simulink model "tests_control_franka"  (R2020b)
settings: Solver=ode1  StartTime=0.0  StopTime=5  FixedStep=0.001  RelTol=1e-4
values from neighbouring files (symbols this model uses):
  a0 = 0.99    [init.m]
  berta = 0.98    [init.m]
  csi = 1    [init.m]
  e_max = 0.01    [init.m]
  F_int_max = 5    [init.m]
  F_max = 2    [init.m]
  M = 1    [init.m]
  mass = 1    [init.m]
  q_max = q_max - deg2rad([0 0 0 10 0 5 0])    [init.m]
  q_min = q_min + deg2rad([0 0 0 10 0 5 0])    [init.m]
libraries: simulink x4
(part 1 of 2)
settings Model: Creator=Rachele  LastModifiedBy=giorg

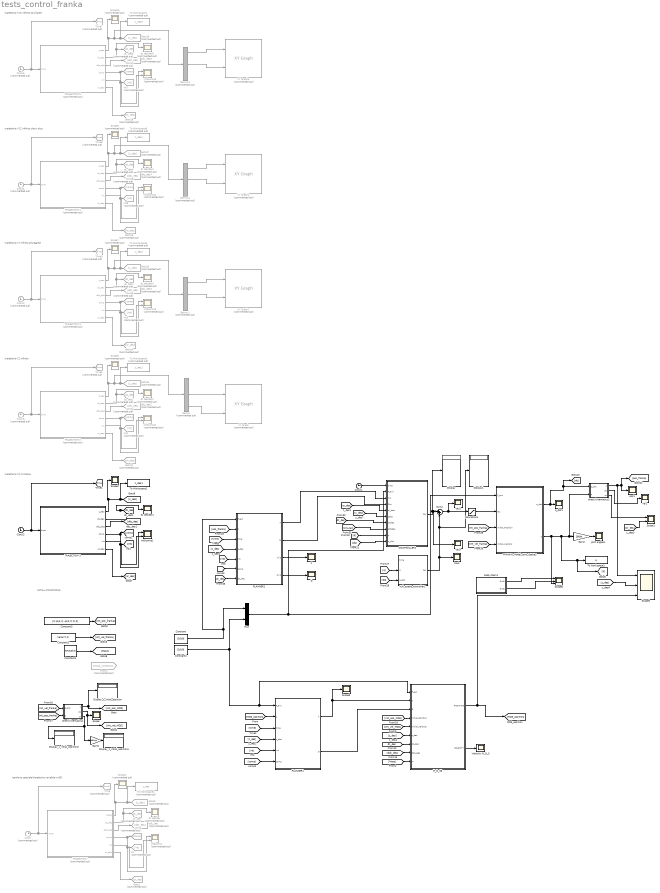
== system tests_control_franka ==
  note: bambino speciale(traiettoria variabile in 6D)
  note: INITIAL CONDITIONS
  note: traiettoria YZ circolare
  note: traiettoria YZ infinito
  note: traiettoria XY infinito allungante
  note: traiettoria XYZ infinito che si alza
  note: traiettoria XYZ infinito oscillante
  CONTROLLER1 : MATLAB Function  TreatAsAtomicUnit=on
  Clock{,3..6} (5 alike) : Clock  Commented=on
  Clock1 : Clock
  Clock2 : Clock
  Constant : Constant  Value=[0;0;0]
  Constant1 : Constant  Value=[0;0;0]
  Constant2 : Constant  Value=zeros(7,1)
  Constant3 : Constant  Value=[0; pi/4; 0; -pi/2; 0; 0; 0]  VectorParams1D=off
  Constant4 : Constant  Value=M*eye(3)
  D : Scope
  Demux{,1..3} (4 alike) : Demux  Commented=on  Outputs=3
  Display : Display
  Display1 : Display
  Display_z_intial_position : Display
  Display_z_intial_position1 : Display
  Display_z_intial_position2 : Display
  FRANKA_Model_Joint_Space2 : Subsystem
  From4 : From  Commented=on  GotoTag=initial_condition
  Gain2 : Gain  Gain=180/pi
  Gain3 : Gain  Gain=180/pi
  Goto{1,12,14,16,18} (5 alike) : Goto  Commented=on  GotoTag=or_des
  Goto{6,13,15,17,19} (5 alike) : Goto  Commented=on  GotoTag=z_des
  Joint angles1 : Scope
  K : Scope
  M_D_S5 : Subsystem
  Mux : Mux  Inputs=2
  PLANNER1 : Subsystem
  PLANNER2 : Subsystem
  Saturation1 : Saturate  UpperLimit=100  LowerLimit=-100
  Scope : Scope
  Scope1 : Scope  NumInputPorts=2
  Scope{4..5,7,9..10} (5 alike) : Scope  Commented=on
  Scope2 : Scope
  Scope3 : Scope
  Scope6 : Scope  NumInputPorts=3
  Scope8 : Scope  NumInputPorts=3
  Subsystem1 : Subsystem
  Sum2 : Sum  Inputs=|++
  TRAJECTORY : Subsystem  Commented=on
  TRAJECTORY1 : Subsystem
  TRAJECTORY2 : Subsystem  Commented=on
  TRAJECTORY3 : Subsystem  Commented=on
  TRAJECTORY4 : Subsystem  Commented=on
  TRAJECTORY5 : Subsystem  Commented=on
  Time{,4..7} (5 alike) : Goto  Commented=on  GotoTag=time
  To Workspace1 : ToWorkspace  VariableName=q  SaveFormat=Timeseries  SampleTime=-1
  To Workspace2 : ToWorkspace  VariableName=z_des1  SaveFormat=Timeseries  SampleTime=-1
      settings: Save2DSignal=2-D array (concatenate along first dimension)
  To Workspace3 : ToWorkspace  Commented=on  VariableName=z_des2  SaveFormat=Timeseries  SampleTime=-1
      settings: Save2DSignal=2-D array (concatenate along first dimension)
  To Workspace4 : ToWorkspace  Commented=on  VariableName=z_des  SaveFormat=Timeseries  SampleTime=-1
      settings: Save2DSignal=2-D array (concatenate along first dimension)
  To Workspace5 : ToWorkspace  Commented=on  VariableName=z_des3  SaveFormat=Timeseries  SampleTime=-1
      settings: Save2DSignal=2-D array (concatenate along first dimension)
  To Workspace6 : ToWorkspace  Commented=on  VariableName=z_des4  SaveFormat=Timeseries  SampleTime=-1
      settings: Save2DSignal=2-D array (concatenate along first dimension)
  To Workspace7 : ToWorkspace  Commented=on  VariableName=z_des5  SaveFormat=Timeseries  SampleTime=-1
      settings: Save2DSignal=2-D array (concatenate along first dimension)
  Velocity M_D_S : Scope
  XY Graph{,1..3} (4 alike) : simulink/Sinks/XY Graph  Commented=on  xmin=-1/2  xmax=1/2  ymin=-1/2  ymax=1/2  st=-1
  comp{,4..7} (5 alike) : Goto  Commented=on  GotoTag=comp
  ddz_des{,2..5} (5 alike) : Goto  Commented=on  GotoTag=ddz_des
  direct kinematics1 : MATLAB Function  TreatAsAtomicUnit=on
  direct kinematics2 : MATLAB Function  TreatAsAtomicUnit=on
  dz desider{,2..5} (5 alike) : Scope  Commented=on
  dz desider1 : Scope
  dz_des{,2..5} (5 alike) : Goto  Commented=on  GotoTag=dz_des  TagVisibility=global
  int{,4..7} (5 alike) : Goto  Commented=on  GotoTag=int
  int&comp{,2..5} (5 alike) : Scope  Commented=on  NumInputPorts=2
  int&comp1 : Scope  NumInputPorts=2
  null_space_controller1 : MATLAB Function  TreatAsAtomicUnit=on
  pos1 : Scope
  q_dot1 : Scope
  tau1 : Scope
  tau2 : Scope
  tau3 : Scope
  vel1 : Scope
  tag scope: dz_des=global
  wires:
  TRAJECTORY/1(z_des) -> Goto6/1, To Workspace4/1, Scope4/1
  [int] -> PLANNER1/5(int)
  PLANNER1/1(K) -> M_D_S5/2(K), Scope3/1
  [init_vel_franka] -> direct kinematics1/1(q_dot)
  Constant3/1 -> [init_pos_franka]
  [MDS_position] -> PLANNER1/2(z)
  Clock/1 -> TRAJECTORY/1(time), Time/1
  [init_vel_MDS] -> M_D_S5/5(Initial_Velocity)
  direct kinematics1/1(z) -> [init_pos_MDS], Display_z_intial_position/1
  Constant4/1 -> [Mass]
  TRAJECTORY/5(int) -> int&comp/2, int/1
  [init_pos_franka] -> direct kinematics1/2(q)
  [dz_des] -> M_D_S5/7(dz_des)
  [z_des] -> PLANNER1/4(z_des)
  [comp] -> PLANNER1/6(comp)
  [ddz_des] -> M_D_S5/8(ddz_des)
  M_D_S5/2(VELOCITY) -> Velocity M_D_S/1
  TRAJECTORY/4(comp) -> int&comp/1, comp/1
  [time] -> PLANNER1/3(time)
  TRAJECTORY/3(ddz_des) -> ddz_des/1
  [Mass] -> M_D_S5/9(M)
  [init_pos_MDS] -> M_D_S5/4(Initial_Position)
  TRAJECTORY/2(dz_des) -> dz desider/1, dz_des/1
  Constant2/1 -> [init_vel_franka]
  [z_des] -> M_D_S5/6(z_des)
  M_D_S5/1(POSITION) -> Scope8/3, [MDS_position]
  [comp] -> PLANNER2/6(comp)
  Subsystem1/1(Out1) -> Scope6/1
  direct kinematics2/3(or) -> Scope1/1
  [or_des] -> CONTROLLER1/5(or_des)
  [dq] -> CONTROLLER1/10(q_dot)
  direct kinematics2/2(dz) -> vel1/1
  [ddz_des] -> CONTROLLER1/8(ddzdes)
  [z_des] -> PLANNER2/4(z_des)
  Gain2/1 -> Joint angles1/1
  [dq] -> null_space_controller1/3(q_dot)
  [time] -> PLANNER2/3(time)
  [pos_franka] -> PLANNER2/2(z)
  [init_pos_franka] -> FRANKA_Model_Joint_Space2/3(Initial_Position)
  FRANKA_Model_Joint_Space2/1(q_dot) -> [dq], direct kinematics2/1(q_dot), q_dot1/1
  direct kinematics2/1(z) -> Scope8/1, pos1/1, [pos_franka]
  [int] -> PLANNER2/5(int)
  [z_des] -> Scope8/2
  [z_des] -> CONTROLLER1/6(zdes)
  null_space_controller1/1(tau) -> tau2/1, Display1/1, Sum2/2
  Sum2/1 -> Saturation1/1, tau1/1
  PLANNER2/1(K) -> CONTROLLER1/3(Km)
  FRANKA_Model_Joint_Space2/2(q) -> Scope6/3, [q], To Workspace1/1, direct kinematics2/2(q), Gain2/1
  [dz_des] -> CONTROLLER1/7(dzdes)
  [q] -> null_space_controller1/2(q)
  PLANNER2/2(D) -> CONTROLLER1/4(Dm)
  [init_vel_franka] -> FRANKA_Model_Joint_Space2/4(Initial_Velocity)
  CONTROLLER1/1(tau) -> Display/1, tau3/1, Sum2/1
  Saturation1/1 -> FRANKA_Model_Joint_Space2/2(tau)
  Subsystem1/2(Out2) -> Scope6/2
  [q] -> CONTROLLER1/9(q)
  PLANNER1/2(D) -> M_D_S5/3(D)
  direct kinematics1/2(dz) -> Scope/1, [init_vel_MDS]
  Gain3/1 -> Display_z_intial_position1/1
  direct kinematics1/3(or) -> Gain3/1, Display_z_intial_position2/1
  PLANNER2/3(kvis) -> K/1
  PLANNER2/4(dvis) -> D/1
  [dz_des] -> PLANNER2/7(dz_des)
  Constant/1 -> Mux/1, PLANNER2/1(F_ext)
  Constant1/1 -> M_D_S5/1(F_ext), PLANNER1/1(F_ext), Mux/2
  Mux/1 -> CONTROLLER1/2(F_ext), FRANKA_Model_Joint_Space2/1(F_ext)
  TRAJECTORY/6(or_des) -> Goto1/1
  Clock1/1 -> CONTROLLER1/1(time)
  [or_des] -> Scope1/2
  TRAJECTORY1/6(or_des) -> [or_des]
  TRAJECTORY1/2(dz_des) -> dz desider1/1, [dz_des]
  TRAJECTORY1/3(ddz_des) -> [ddz_des]
  TRAJECTORY1/4(comp) -> [comp], int&comp1/1
  TRAJECTORY1/5(int) -> [int], int&comp1/2
  Clock2/1 -> [time], TRAJECTORY1/1(time)
  TRAJECTORY1/1(z_des) -> Scope2/1, To Workspace2/1, [z_des]
  Clock3/1 -> Time4/1, TRAJECTORY2/1(time)
  TRAJECTORY2/1(z_des) -> Scope5/1, Demux/1, To Workspace3/1, Goto13/1
  TRAJECTORY2/5(int) -> int4/1, int&comp2/2
  TRAJECTORY2/4(comp) -> comp4/1, int&comp2/1
  TRAJECTORY2/6(or_des) -> Goto12/1
  TRAJECTORY2/2(dz_des) -> dz_des2/1, dz desider2/1
  TRAJECTORY2/3(ddz_des) -> ddz_des2/1
  Demux/2 -> XY Graph/1
  Demux/3 -> XY Graph/2
  TRAJECTORY3/3(ddz_des) -> ddz_des3/1
  TRAJECTORY3/2(dz_des) -> dz_des3/1, dz desider3/1
  TRAJECTORY3/6(or_des) -> Goto14/1
  TRAJECTORY3/4(comp) -> comp5/1, int&comp3/1
  TRAJECTORY3/1(z_des) -> Scope7/1, Demux1/1, To Workspace5/1, Goto15/1
  TRAJECTORY3/5(int) -> int5/1, int&comp3/2
  Clock4/1 -> Time5/1, TRAJECTORY3/1(time)
  Demux1/1 -> XY Graph1/1
  Demux1/2 -> XY Graph1/2
  Demux2/2 -> XY Graph2/2
  Demux2/1 -> XY Graph2/1
  Clock5/1 -> TRAJECTORY4/1(time), Time6/1
  TRAJECTORY4/5(int) -> int&comp4/2, int6/1
  TRAJECTORY4/1(z_des) -> Goto17/1, To Workspace6/1, Demux2/1, Scope9/1
  TRAJECTORY4/4(comp) -> int&comp4/1, comp6/1
  TRAJECTORY4/6(or_des) -> Goto16/1
  TRAJECTORY4/2(dz_des) -> dz desider4/1, dz_des4/1
  TRAJECTORY4/3(ddz_des) -> ddz_des4/1
  TRAJECTORY5/3(ddz_des) -> ddz_des5/1
  TRAJECTORY5/5(int) -> int&comp5/2, int7/1
  TRAJECTORY5/6(or_des) -> Goto18/1
  TRAJECTORY5/4(comp) -> int&comp5/1, comp7/1
  Demux3/1 -> XY Graph3/1
  TRAJECTORY5/1(z_des) -> Goto19/1, To Workspace7/1, Demux3/1, Scope10/1
  TRAJECTORY5/2(dz_des) -> dz desider5/1, dz_des5/1
  Demux3/2 -> XY Graph3/2
  Clock6/1 -> TRAJECTORY5/1(time), Time7/1

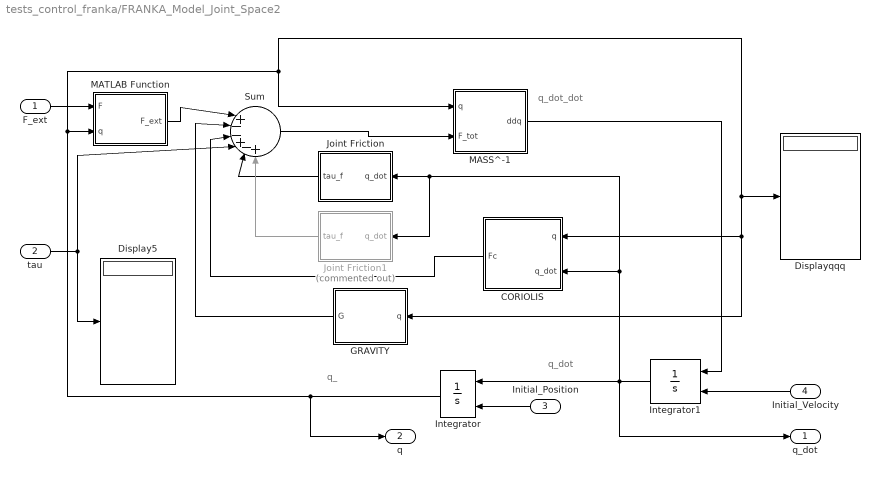
== system tests_control_franka/FRANKA_Model_Joint_Space2 ==
  note: q_dot
  note: q_dot_dot
  note: q_
  F_ext : Inport
  tau : Inport  Port=2
  Initial_Position : Inport  Port=3
  Initial_Velocity : Inport  Port=4
  CORIOLIS : MATLAB Function  TreatAsAtomicUnit=on
  Display5 : Display
  Displayqqq : Display
  GRAVITY : MATLAB Function  TreatAsAtomicUnit=on
  Integrator : Integrator  InitialConditionSource=external
  Integrator1 : Integrator  InitialConditionSource=external  InitialCondition=[0;0]
  Joint Friction : MATLAB Function  TreatAsAtomicUnit=on
  Joint Friction1 : MATLAB Function  Commented=on  TreatAsAtomicUnit=on
  MASS^-1 : MATLAB Function  TreatAsAtomicUnit=on
  MATLAB Function : MATLAB Function  TreatAsAtomicUnit=on
  Sum : Sum  Inputs=||+--+-+
  q_dot : Outport
  q : Outport  Port=2
  wires:
  GRAVITY/1(G) -> Sum/2
  MATLAB Function/1(F_ext) -> Sum/1
  Initial_Position/1 -> Integrator/2
  F_ext/1 -> MATLAB Function/1(F)
  Integrator/1 -> MASS^-1/1(q), GRAVITY/1(q), CORIOLIS/1(q), Displayqqq/1, MATLAB Function/2(q), q/1
  Integrator1/1 -> q_dot/1, CORIOLIS/2(q_dot), Joint Friction1/1(q_dot), Joint Friction/1(q_dot), Integrator/1
  Initial_Velocity/1 -> Integrator1/2
  MASS^-1/1(ddq) -> Integrator1/1
  Sum/1 -> MASS^-1/2(F_tot)
  CORIOLIS/1(Fc) -> Sum/3
  tau/1 -> Display5/1, Sum/4
  Joint Friction/1(tau_f) -> Sum/5
  Joint Friction1/1(tau_f) -> Sum/6

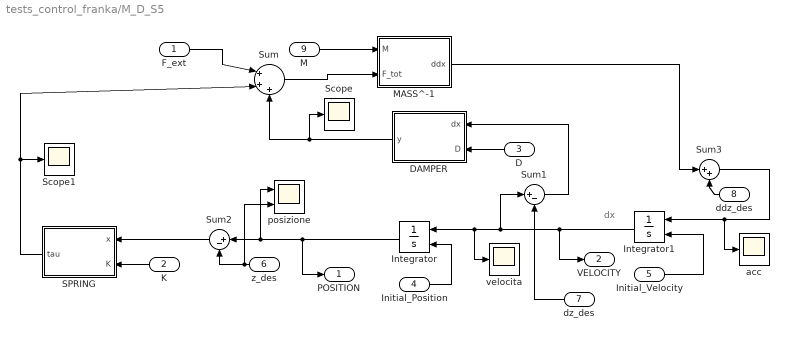
== system tests_control_franka/M_D_S5 ==
  note: dx
  F_ext : Inport
  K : Inport  Port=2
  D : Inport  Port=3
  Initial_Position : Inport  Port=4
  Initial_Velocity : Inport  Port=5
  z_des : Inport  Port=6
  dz_des : Inport  Port=7
  ddz_des : Inport  Port=8
  M : Inport  Port=9
  DAMPER : MATLAB Function  TreatAsAtomicUnit=on
  Integrator : Integrator  InitialConditionSource=external
  Integrator1 : Integrator  InitialConditionSource=external
  MASS^-1 : MATLAB Function  TreatAsAtomicUnit=on
  SPRING : MATLAB Function  TreatAsAtomicUnit=on
  Scope : Scope
  Scope1 : Scope
  Sum : Sum  Inputs=|+++
  Sum1 : Sum  Inputs=|+-
  Sum2 : Sum  Inputs=|+-
  Sum3 : Sum  Inputs=|++
  acc : Scope
  posizione : Scope  NumInputPorts=2
  velocita : Scope
  POSITION : Outport
  VELOCITY : Outport  Port=2
  wires:
  Integrator1/1 -> velocita/1, Integrator/1, Sum1/1, VELOCITY/1
  SPRING/1(tau) -> Sum/2, Scope1/1
  Integrator/1 -> posizione/1, Sum2/1, POSITION/1
  DAMPER/1(y) -> Scope/1, Sum/3
  Sum/1 -> MASS^-1/2(F_tot)
  M/1 -> MASS^-1/1(M)
  D/1 -> DAMPER/2(D)
  K/1 -> SPRING/2(K)
  Initial_Velocity/1 -> Integrator1/2
  Initial_Position/1 -> Integrator/2
  z_des/1 -> posizione/2, Sum2/2
  Sum2/1 -> SPRING/1(x)
  MASS^-1/1(ddx) -> Sum3/1
  Sum1/1 -> DAMPER/1(dx)
  Sum3/1 -> acc/1, Integrator1/1
  dz_des/1 -> Sum1/2
  ddz_des/1 -> Sum3/2
  F_ext/1 -> Sum/1

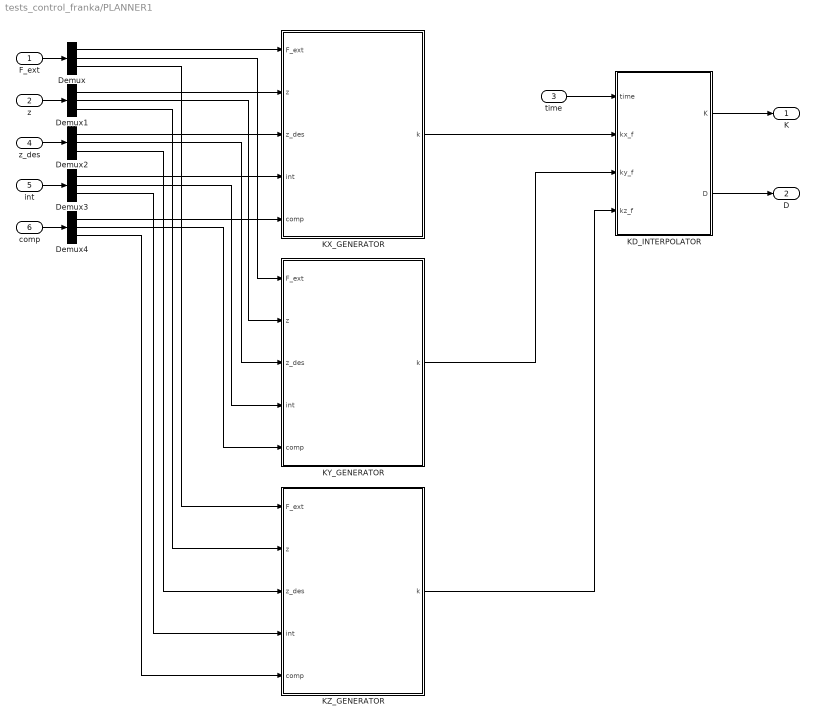
== system tests_control_franka/PLANNER1 ==
  F_ext : Inport
  z : Inport  Port=2
  time : Inport  Port=3
  z_des : Inport  Port=4
  int : Inport  Port=5
  comp : Inport  Port=6
  Demux{,1..4} (5 alike) : Demux  Outputs=3
  "KD_INTERPOLATOR " : MATLAB Function  TreatAsAtomicUnit=on
  KX_GENERATOR : MATLAB Function  TreatAsAtomicUnit=on
  KY_GENERATOR : MATLAB Function  TreatAsAtomicUnit=on
  KZ_GENERATOR : MATLAB Function  TreatAsAtomicUnit=on
  K : Outport
  D : Outport  Port=2
  wires:
  KZ_GENERATOR/1(k) -> "KD_INTERPOLATOR "/4(kz_f)
  KY_GENERATOR/1(k) -> "KD_INTERPOLATOR "/3(ky_f)
  Demux4/3 -> KZ_GENERATOR/5(comp)
  Demux3/3 -> KZ_GENERATOR/4(int)
  Demux2/3 -> KZ_GENERATOR/3(z_des)
  Demux1/3 -> KZ_GENERATOR/2(z)
  Demux/3 -> KZ_GENERATOR/1(F_ext)
  Demux4/2 -> KY_GENERATOR/5(comp)
  Demux3/2 -> KY_GENERATOR/4(int)
  Demux2/2 -> KY_GENERATOR/3(z_des)
  Demux1/2 -> KY_GENERATOR/2(z)
  Demux/2 -> KY_GENERATOR/1(F_ext)
  comp/1 -> Demux4/1
  int/1 -> Demux3/1
  z_des/1 -> Demux2/1
  z/1 -> Demux1/1
  F_ext/1 -> Demux/1
  Demux4/1 -> KX_GENERATOR/5(comp)
  Demux3/1 -> KX_GENERATOR/4(int)
  Demux2/1 -> KX_GENERATOR/3(z_des)
  Demux1/1 -> KX_GENERATOR/2(z)
  Demux/1 -> KX_GENERATOR/1(F_ext)
  KX_GENERATOR/1(k) -> "KD_INTERPOLATOR "/2(kx_f)
  "KD_INTERPOLATOR "/1(K) -> K/1
  "KD_INTERPOLATOR "/2(D) -> D/1
  time/1 -> "KD_INTERPOLATOR "/1(time)

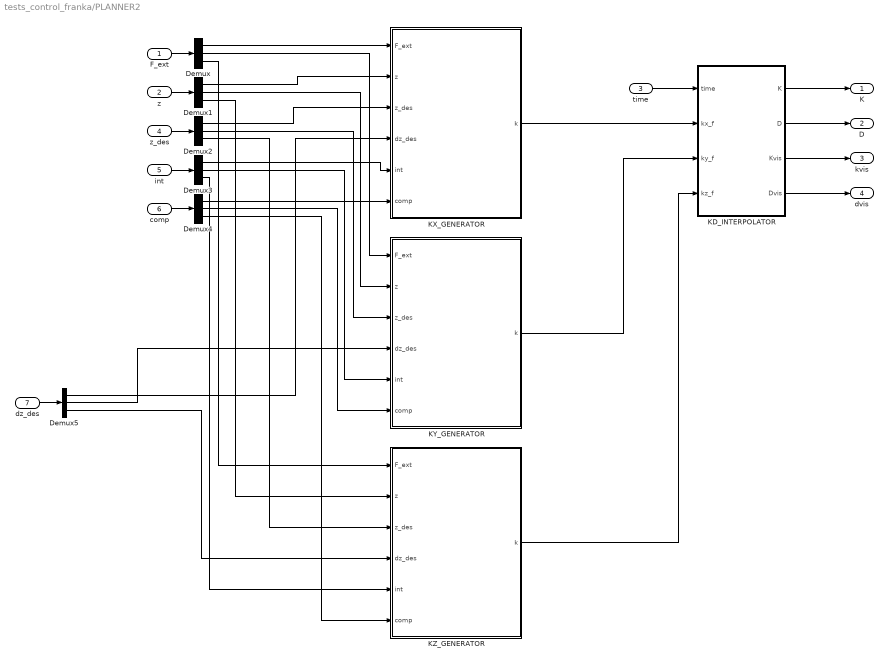
== system tests_control_franka/PLANNER2 ==
  F_ext : Inport
  z : Inport  Port=2
  time : Inport  Port=3
  z_des : Inport  Port=4
  int : Inport  Port=5
  comp : Inport  Port=6
  dz_des : Inport  Port=7
  Demux{,1..5} (6 alike) : Demux  Outputs=3
  "KD_INTERPOLATOR " : MATLAB Function  TreatAsAtomicUnit=on
  KX_GENERATOR : MATLAB Function  TreatAsAtomicUnit=on
  KY_GENERATOR : MATLAB Function  TreatAsAtomicUnit=on
  KZ_GENERATOR : MATLAB Function  TreatAsAtomicUnit=on
  K : Outport
  D : Outport  Port=2
  kvis : Outport  Port=3
  dvis : Outport  Port=4
  wires:
  time/1 -> "KD_INTERPOLATOR "/1(time)
  "KD_INTERPOLATOR "/2(D) -> D/1
  "KD_INTERPOLATOR "/1(K) -> K/1
  KX_GENERATOR/1(k) -> "KD_INTERPOLATOR "/2(kx_f)
  Demux/1 -> KX_GENERATOR/1(F_ext)
  Demux1/1 -> KX_GENERATOR/2(z)
  Demux2/1 -> KX_GENERATOR/3(z_des)
  Demux3/1 -> KX_GENERATOR/5(int)
  Demux4/1 -> KX_GENERATOR/6(comp)
  F_ext/1 -> Demux/1
  z/1 -> Demux1/1
  z_des/1 -> Demux2/1
  int/1 -> Demux3/1
  comp/1 -> Demux4/1
  Demux/2 -> KY_GENERATOR/1(F_ext)
  Demux1/2 -> KY_GENERATOR/2(z)
  Demux2/2 -> KY_GENERATOR/3(z_des)
  Demux3/2 -> KY_GENERATOR/5(int)
  Demux4/2 -> KY_GENERATOR/6(comp)
  Demux/3 -> KZ_GENERATOR/1(F_ext)
  Demux1/3 -> KZ_GENERATOR/2(z)
  Demux2/3 -> KZ_GENERATOR/3(z_des)
  Demux3/3 -> KZ_GENERATOR/5(int)
  Demux4/3 -> KZ_GENERATOR/6(comp)
  KY_GENERATOR/1(k) -> "KD_INTERPOLATOR "/3(ky_f)
  KZ_GENERATOR/1(k) -> "KD_INTERPOLATOR "/4(kz_f)
  "KD_INTERPOLATOR "/3(Kvis) -> kvis/1
  "KD_INTERPOLATOR "/4(Dvis) -> dvis/1
  dz_des/1 -> Demux5/1
  Demux5/3 -> KZ_GENERATOR/4(dz_des)
  Demux5/1 -> KX_GENERATOR/4(dz_des)
  Demux5/2 -> KY_GENERATOR/4(dz_des)

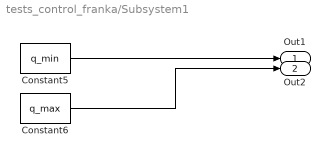
== system tests_control_franka/Subsystem1 ==
  Constant5 : Constant  Value=q_min
  Constant6 : Constant  Value=q_max
  Out1 : Outport
  Out2 : Outport  Port=2
  wires:
  Constant5/1 -> Out1/1
  Constant6/1 -> Out2/1

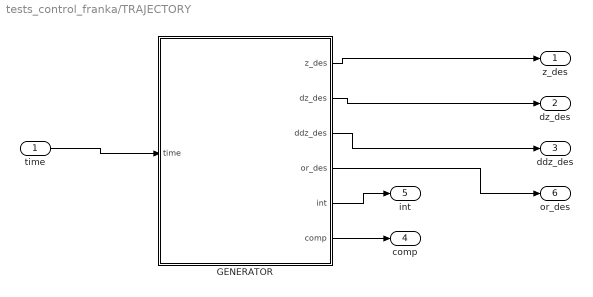
== system tests_control_franka/TRAJECTORY ==
  time : Inport
  GENERATOR : MATLAB Function  TreatAsAtomicUnit=on
  z_des : Outport
  dz_des : Outport  Port=2
  ddz_des : Outport  Port=3
  comp : Outport  Port=4
  int : Outport  Port=5
  or_des : Outport  Port=6
  wires:
  GENERATOR/1(z_des) -> z_des/1
  GENERATOR/2(dz_des) -> dz_des/1
  GENERATOR/3(ddz_des) -> ddz_des/1
  GENERATOR/5(int) -> int/1
  GENERATOR/6(comp) -> comp/1
  time/1 -> GENERATOR/1(time)
  GENERATOR/4(or_des) -> or_des/1

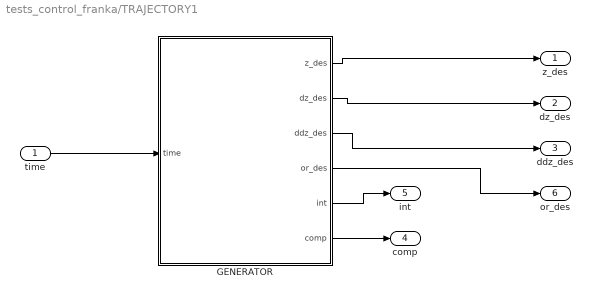
== system tests_control_franka/TRAJECTORY1 ==
  time : Inport
  GENERATOR : MATLAB Function  TreatAsAtomicUnit=on
  z_des : Outport
  dz_des : Outport  Port=2
  ddz_des : Outport  Port=3
  comp : Outport  Port=4
  int : Outport  Port=5
  or_des : Outport  Port=6
  wires:
  GENERATOR/4(or_des) -> or_des/1
  time/1 -> GENERATOR/1(time)
  GENERATOR/6(comp) -> comp/1
  GENERATOR/5(int) -> int/1
  GENERATOR/3(ddz_des) -> ddz_des/1
  GENERATOR/2(dz_des) -> dz_des/1
  GENERATOR/1(z_des) -> z_des/1

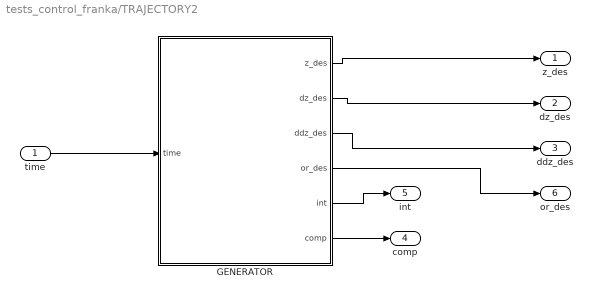
== system tests_control_franka/TRAJECTORY2 ==
  time : Inport
  GENERATOR : MATLAB Function  TreatAsAtomicUnit=on
  z_des : Outport
  dz_des : Outport  Port=2
  ddz_des : Outport  Port=3
  comp : Outport  Port=4
  int : Outport  Port=5
  or_des : Outport  Port=6
  wires:
  GENERATOR/4(or_des) -> or_des/1
  time/1 -> GENERATOR/1(time)
  GENERATOR/6(comp) -> comp/1
  GENERATOR/5(int) -> int/1
  GENERATOR/3(ddz_des) -> ddz_des/1
  GENERATOR/2(dz_des) -> dz_des/1
  GENERATOR/1(z_des) -> z_des/1

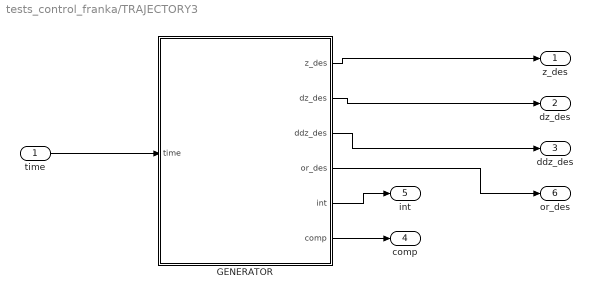
== system tests_control_franka/TRAJECTORY3 ==
  time : Inport
  GENERATOR : MATLAB Function  TreatAsAtomicUnit=on
  z_des : Outport
  dz_des : Outport  Port=2
  ddz_des : Outport  Port=3
  comp : Outport  Port=4
  int : Outport  Port=5
  or_des : Outport  Port=6
  wires:
  GENERATOR/4(or_des) -> or_des/1
  time/1 -> GENERATOR/1(time)
  GENERATOR/6(comp) -> comp/1
  GENERATOR/5(int) -> int/1
  GENERATOR/3(ddz_des) -> ddz_des/1
  GENERATOR/2(dz_des) -> dz_des/1
  GENERATOR/1(z_des) -> z_des/1

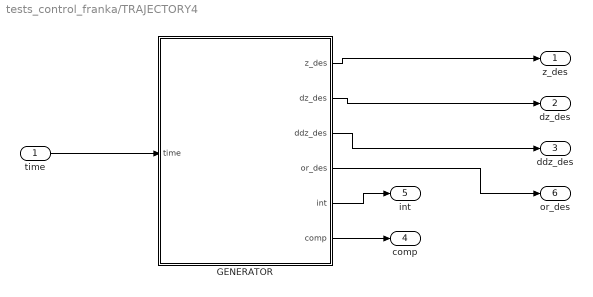
== system tests_control_franka/TRAJECTORY4 ==
  time : Inport
  GENERATOR : MATLAB Function  TreatAsAtomicUnit=on
  z_des : Outport
  dz_des : Outport  Port=2
  ddz_des : Outport  Port=3
  comp : Outport  Port=4
  int : Outport  Port=5
  or_des : Outport  Port=6
  wires:
  GENERATOR/1(z_des) -> z_des/1
  GENERATOR/2(dz_des) -> dz_des/1
  GENERATOR/3(ddz_des) -> ddz_des/1
  GENERATOR/5(int) -> int/1
  GENERATOR/6(comp) -> comp/1
  time/1 -> GENERATOR/1(time)
  GENERATOR/4(or_des) -> or_des/1

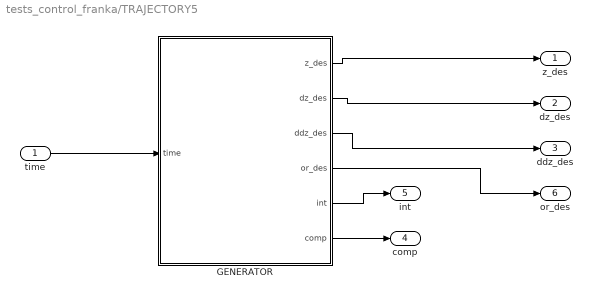
== system tests_control_franka/TRAJECTORY5 ==
  time : Inport
  GENERATOR : MATLAB Function  TreatAsAtomicUnit=on
  z_des : Outport
  dz_des : Outport  Port=2
  ddz_des : Outport  Port=3
  comp : Outport  Port=4
  int : Outport  Port=5
  or_des : Outport  Port=6
  wires:
  GENERATOR/1(z_des) -> z_des/1
  GENERATOR/2(dz_des) -> dz_des/1
  GENERATOR/3(ddz_des) -> ddz_des/1
  GENERATOR/5(int) -> int/1
  GENERATOR/6(comp) -> comp/1
  time/1 -> GENERATOR/1(time)
  GENERATOR/4(or_des) -> or_des/1

== matlab function tests_control_franka/PLANNER1/KX_GENERATOR ==
  settings: updateMethod=DISCRETE  sampleTime=Ts
  data: k output; F_ext input; z input; z_des input; int input; comp input; e_max parameter; F_max parameter; F_int_max parameter
function k = fcn(F_ext, z, z_des, int, comp, e_max, F_max, F_int_max)
%% Description
% Set the K coefficient for a variable impedance controller based on a
% desired trajectory

%% Outputs
% k             stiffness

%% Inputs
% F_ext         measured external force
% z_des         desired trajectory
% z             current position
% int, comp     booleans for the interaction and compensation phase

%% Parameters
% F_int_max     desired interaction force
% F_max         nominal disturbance forces
% e_max         maximum steady-state error

%% persistent initialization
persistent ki kc F_comp int_prec comp_prec z_int z_int_dir 
if isempty(ki)
   ki = F_max/e_max;        % k obtained from interaction
end
if isempty(F_comp)
   F_comp = 0;              % weight to compensate
end
if isempty(kc)
      kc = F_max/e_max;     % k obtained from compensation
end
if isempty(z_int) 
    z_int = 1000;       % obstacle(or interaction) position
end
if isempty(z_int_dir) 
    z_int_dir = 0;          % prohibited direction due to the obstacle
end
if isempty(int_prec)
    int_prec = 0;           % previous values of int
end
if isempty(comp_prec)
    comp_prec = 0;          % previous values od comp
end

%% INTERACTION
% set ki in order to match a desired interaction force with the
% envirorment, and store interaction's position when detected
% X axes
if int == 1
    % detection of an interaction 
    if abs(F_ext-F_comp) > F_max
        if z_int == 1000                     % z_int has not been set yet
            z_int = z;
            z_int_dir = -sign(F_ext-F_comp);
        end
    end
    % setting of ki
    if abs(F_ext-F_comp) > F_int_max 
        % if interaction force is higher than threshold
        if ki*abs(z-z_des) > F_int_max
            ktemp_x = F_int_max/abs(z-z_des);
            if ktemp_x < ki                % ki needs to be only decreased
                ki = ktemp_x;
            end
        end
    end
end

%% COMPENSATION
% set kc in order to compensate the effect of the weight of the object,
% and store it
% X axes
if comp == 1
    % compensation detection
    if z_int == 1000                     % z_int not set before
       if abs(F_ext)/kc > e_max         
            kc = abs(F_ext)/e_max;
            F_comp = F_ext;
       end
    else 
        if z_int_dir == 1                % obstacle in above
            if z < z_int
                if abs(F_ext)/kc > e_max 
                    kc = abs(F_ext)/e_max;
                    F_comp = F_ext;
                end
            end
        else                                % obstacle is below
            if z > z_int
                if abs(F_ext)/kc > e_max
                    kc = abs(F_ext)/e_max;
                    F_comp = F_ext;
                end
            end
        end 
   end
end

%% reset to default values when comp or int shifts to zero
if comp==0 && comp_prec==1
    kc = F_max/e_max;
    F_comp = 0;
end
if int==0 && int_prec==1
    ki = F_max/e_max;
end

%% from int to comp and vice versa
if int==1 && int_prec==0
    if comp_prec == 1
        ki = kc;
    end
    z_int=1000;
    z_int_dir=0;
end
if comp == 1 && comp_prec==0
    if int_prec == 1
        kc = ki;
    end
end

% update to last booleans
int_prec = int;
comp_prec = comp;


%% Selection of Final Values of D-K
% default values
k = abs(F_max)/e_max;

% compensation
if comp == 1
    k = kc;
end

% both compensation and interaction are activated
% if "away" from obstacle set k = kc else ki
if int == 1
    k = ki;
    if comp == 1
        if z_int == 1000
            k = kc;                       % obstacle not reached
        else
            if z_int_dir == 1
                if z_des < z_int
                    k = kc;               % obstacle reached but "going away"
                end
            else
                if z_des > z_int
                    k = kc;               % obstacle reached but "going away"
                end
            end
        end
    else
        if z_int == 1000
            k = F_max/e_max;            % restore to default
        else
            if z_int_dir == 1
                if z_des < z_int
                    k = F_max/e_max;    % restore because "going away"
                end
            else
                if z_des > z_int
                    k = F_max/e_max;    % restore because "going away"
                end
            end
        end
    end
end

end

== matlab function tests_control_franka/PLANNER1/KY_GENERATOR ==
  settings: updateMethod=DISCRETE  sampleTime=Ts
  data: k output; F_ext input; z input; z_des input; int input; comp input; e_max parameter; F_max parameter; F_int_max parameter
function k = fcn(F_ext, z, z_des, int, comp, e_max, F_max, F_int_max)
%% Description
% Set the K coefficient for a variable impedance controller based on a
% desired trajectory

%% Outputs
% k             stiffness

%% Inputs
% F_ext         measured external force
% z_des         desired trajectory
% z             current position
% int, comp     booleans for the interaction and compensation phase

%% Parameters
% F_int_max     desired interaction force
% F_max         nominal disturbance forces
% e_max         maximum steady-state error

%% persistent initialization
persistent ki kc F_comp int_prec comp_prec z_int z_int_dir 
if isempty(ki)
   ki = F_max/e_max;        % k obtained from interaction
end
if isempty(F_comp)
   F_comp = 0;              % weight to compensate
end
if isempty(kc)
      kc = F_max/e_max;     % k obtained from compensation
end
if isempty(z_int) 
    z_int = 1000;       % obstacle(or interaction) position
end
if isempty(z_int_dir) 
    z_int_dir = 0;          % prohibited direction due to the obstacle
end
if isempty(int_prec)
    int_prec = 0;           % previous values of int
end
if isempty(comp_prec)
    comp_prec = 0;          % previous values od comp
end

%% INTERACTION
% set ki in order to match a desired interaction force with the
% envirorment, and store interaction's position when detected
% X axes
if int == 1
    % detection of an interaction 
    if abs(F_ext-F_comp) > F_max
        if z_int == 1000                     % z_int has not been set yet
            z_int = z;
            z_int_dir = -sign(F_ext-F_comp);
        end
    end
    % setting of ki
    if abs(F_ext-F_comp) > F_int_max 
        % if interaction force is higher than threshold
        if ki*abs(z-z_des) > F_int_max
            ktemp_x = F_int_max/abs(z-z_des);
            if ktemp_x < ki                % ki needs to be only decreased
                ki = ktemp_x;
            end
        end
    end
end

%% COMPENSATION
% set kc in order to compensate the effect of the weight of the object,
% and store it
% X axes
if comp == 1
    % compensation detection
    if z_int == 1000                     % z_int not set before
       if abs(F_ext)/kc > e_max         
            kc = abs(F_ext)/e_max;
            F_comp = F_ext;
       end
    else 
        if z_int_dir == 1                % obstacle in above
            if z < z_int
                if abs(F_ext)/kc > e_max 
                    kc = abs(F_ext)/e_max;
                    F_comp = F_ext;
                end
            end
        else                                % obstacle is below
            if z > z_int
                if abs(F_ext)/kc > e_max
                    kc = abs(F_ext)/e_max;
                    F_comp = F_ext;
                end
            end
        end 
   end
end

%% reset to default values when comp or int shifts to zero
if comp==0 && comp_prec==1
    kc = F_max/e_max;
    F_comp = 0;
end
if int==0 && int_prec==1
    ki = F_max/e_max;
end

%% from int to comp and vice versa
if int==1 && int_prec==0
    if comp_prec == 1
        ki = kc;
    end
    z_int=1000;
    z_int_dir=0;
end
if comp == 1 && comp_prec==0
    if int_prec == 1
        kc = ki;
    end
end

% update to last booleans
int_prec = int;
comp_prec = comp;


%% Selection of Final Values of D-K
% default values
k = abs(F_max)/e_max;

% compensation
if comp == 1
    k = kc;
end

% both compensation and interaction are activated
% if "away" from obstacle set k = kc else ki
if int == 1
    k = ki;
    if comp == 1
        if z_int == 1000
            k = kc;                       % obstacle not reached
        else
            if z_int_dir == 1
                if z_des < z_int
                    k = kc;               % obstacle reached but "going away"
                end
            else
                if z_des > z_int
                    k = kc;               % obstacle reached but "going away"
                end
            end
        end
    else
        if z_int == 1000
            k = F_max/e_max;            % restore to default
        else
            if z_int_dir == 1
                if z_des < z_int
                    k = F_max/e_max;    % restore because "going away"
                end
            else
                if z_des > z_int
                    k = F_max/e_max;    % restore because "going away"
                end
            end
        end
    end
end

end

== matlab function tests_control_franka/TRAJECTORY/GENERATOR ==
  data: time input; z_des output; dz_des output; ddz_des output; or_des output; int output; comp output
function  [z_des, dz_des, ddz_des, or_des, int, comp] = fcn(time)
coder.extrinsic('wrapToPi')
t= time;
int = [0; 0; 0];
comp = [0; 0; 0];
q = [0; pi/4; 0; -pi/2; 0; 0; 0];
or_init = [-3.14;0.7;0];
pos_init = [0.35; 0; 0.3];
or_des = or_init + [pi/4*sin(t);pi/4*sin(t);pi/4*(1+sin(t))];
or_des = wrapToPi(or_des);
%or_des = [-3.14;0.7;0];

z_des = pos_init + [cos(t)/8; cos(2*t)/4; sin(2*t)/4];
dz_des = [-sin(t)/4; -sin(2*t)/2; cos(2*t)/2];
ddz_des = [-cos(t)/2; -cos(2*t); -sin(2*t)];

end

== matlab function tests_control_franka/PLANNER1/KZ_GENERATOR ==
  settings: updateMethod=DISCRETE  sampleTime=Ts
  data: k output; F_ext input; z input; z_des input; int input; comp input; e_max parameter; F_max parameter; F_int_max parameter
function k = fcn(F_ext, z, z_des, int, comp, e_max, F_max, F_int_max)
%% Description
% Set the K coefficient for a variable impedance controller based on a
% desired trajectory

%% Outputs
% k             stiffness

%% Inputs
% F_ext         measured external force
% z_des         desired trajectory
% z             current position
% int, comp     booleans for the interaction and compensation phase

%% Parameters
% F_int_max     desired interaction force
% F_max         nominal disturbance forces
% e_max         maximum steady-state error

%% persistent initialization
persistent ki kc F_comp int_prec comp_prec z_int z_int_dir 
if isempty(ki)
   ki = F_max/e_max;        % k obtained from interaction
end
if isempty(F_comp)
   F_comp = 0;              % weight to compensate
end
if isempty(kc)
      kc = F_max/e_max;     % k obtained from compensation
end
if isempty(z_int) 
    z_int = 1000;       % obstacle(or interaction) position
end
if isempty(z_int_dir) 
    z_int_dir = 0;          % prohibited direction due to the obstacle
end
if isempty(int_prec)
    int_prec = 0;           % previous values of int
end
if isempty(comp_prec)
    comp_prec = 0;          % previous values od comp
end

%% INTERACTION
% set ki in order to match a desired interaction force with the
% envirorment, and store interaction's position when detected
% X axes
if int == 1
    % detection of an interaction 
    if abs(F_ext-F_comp) > F_max
        if z_int == 1000                     % z_int has not been set yet
            z_int = z;
            z_int_dir = -sign(F_ext-F_comp);
        end
    end
    % setting of ki
    if abs(F_ext-F_comp) > F_int_max 
        % if interaction force is higher than threshold
        if ki*abs(z-z_des) > F_int_max
            ktemp_x = F_int_max/abs(z-z_des);
            if ktemp_x < ki                % ki needs to be only decreased
                ki = ktemp_x;
            end
        end
    end
end

%% COMPENSATION
% set kc in order to compensate the effect of the weight of the object,
% and store it
% X axes
if comp == 1
    % compensation detection
    if z_int == 1000                     % z_int not set before
       if abs(F_ext)/kc > e_max         
            kc = abs(F_ext)/e_max;
            F_comp = F_ext;
       end
    else 
        if z_int_dir == 1                % obstacle in above
            if z < z_int
                if abs(F_ext)/kc > e_max 
                    kc = abs(F_ext)/e_max;
                    F_comp = F_ext;
                end
            end
        else                                % obstacle is below
            if z > z_int
                if abs(F_ext)/kc > e_max
                    kc = abs(F_ext)/e_max;
                    F_comp = F_ext;
                end
            end
        end 
   end
end

%% reset to default values when comp or int shifts to zero
if comp==0 && comp_prec==1
    kc = F_max/e_max;
    F_comp = 0;
end
if int==0 && int_prec==1
    ki = F_max/e_max;
end

%% from int to comp and vice versa
if int==1 && int_prec==0
    if comp_prec == 1
        ki = kc;
    end
    z_int=1000;
    z_int_dir=0;
end
if comp == 1 && comp_prec==0
    if int_prec == 1
        kc = ki;
    end
end

% update to last booleans
int_prec = int;
comp_prec = comp;


%% Selection of Final Values of D-K
% default values
k = abs(F_max)/e_max;

% compensation
if comp == 1
    k = kc;
end

% both compensation and interaction are activated
% if "away" from obstacle set k = kc else ki
if int == 1
    k = ki;
    if comp == 1
        if z_int == 1000
            k = kc;                       % obstacle not reached
        else
            if z_int_dir == 1
                if z_des < z_int
                    k = kc;               % obstacle reached but "going away"
                end
            else
                if z_des > z_int
                    k = kc;               % obstacle reached but "going away"
                end
            end
        end
    else
        if z_int == 1000
            k = F_max/e_max;            % restore to default
        else
            if z_int_dir == 1
                if z_des < z_int
                    k = F_max/e_max;    % restore because "going away"
                end
            else
                if z_des > z_int
                    k = F_max/e_max;    % restore because "going away"
                end
            end
        end
    end
end

end

== matlab function tests_control_franka/direct kinematics1 ==
  data: q_dot input double; q input double; z output double; dz output double; or output
function [z,dz,or] = fcn(q_dot,q)
coder.extrinsic('get_Ja');
% persistent dh_c
% if isempty(dh_c)
%     dh_c = Load_Franka_DH();
% end
[DH, Conv] = Load_Franka_DH();
z = zeros(3,1);
%z = get_pos(q);

[p,R] = DirectKinematic(DH,[q;0],Conv);
z = p;
phi = atan2(R(2,1),R(1,1));
teta = atan2(-R(3,1),sqrt(R(3,2)^2 + R(3,3)^2)); 
psi = atan2(R(3,2),R(3,3));
or = [phi teta psi]';

Ja = zeros(6,7);
Ja = get_Ja(q);

dz = zeros(3,1);
dz = Ja(1:3,1:7)*q_dot;

end

== matlab function tests_control_franka/M_D_S5/DAMPER ==
  data: dx input; y output; D input
function y = fcn(dx, D)
y = - D*dx;
end

== matlab function tests_control_franka/M_D_S5/MASS^-1 ==
  data: M input; ddx output; F_tot input
function ddx = fcn(M,F_tot)
ddx = (M^-1)*F_tot;
end

== matlab function tests_control_franka/M_D_S5/SPRING ==
  data: x input; tau output; K input
function tau = fcn(x, K)
tau= -K*x;
end

== matlab function tests_control_franka/CONTROLLER1 ==
  settings: updateMethod=DISCRETE  sampleTime=Ts
  data: time input; F_ext input; Km input; Dm input; or_des input; zdes input; tau output double; dzdes input; ddzdes input; q input; q_dot input; M parameter
function tau = fcn(time, F_ext, Km, Dm, or_des, zdes, dzdes, ddzdes, q, q_dot, M)
coder.extrinsic('get_MassMatrix','get_Ja_dot','get_Ja','get_GravityVector','get_FrictionTorque','get_CoriolisMatrix')
coder.extrinsic('wrapToPi')
% dz = zeros(2,1);
% z = zeros(2,1);
B = zeros(7,7);
S = zeros(7,7);
G = zeros(7,1);
Ja = zeros(6,7);
Ja_dot = zeros(6,7);
tau_fric = zeros(7,1);
Bm = eye(6)*M;
Ja = get_Ja(q);
Ja_dot = get_Ja_dot(q,q_dot);
%Ja_dot(4:6,:) = zeros(3, 7);
Ja(isnan(Ja)) = 0;
Ja_dot(isnan(Ja_dot)) = 0;
%% Computation of end-effector's position and orientation 
[DH, Conv] = Load_Franka_DH();
[p,R] = DirectKinematic(DH,[q;0],Conv);
z = zeros(3,1);
z = p;
dz = Ja(1:3,1:7)*q_dot;
phi = atan2(R(2,1),R(1,1));
teta = atan2(-R(3,1),sqrt(R(3,2)^2 + R(3,3)^2)); 
psi = atan2(R(3,2),R(3,3));
or = [phi teta psi]';
% pseudoinverse
B = get_MassMatrix(q);
Ja_inv = inv(B)*(Ja')*inv(Ja*inv(B)*Ja');
%Ja_inv = (Ja')*inv(Ja*Ja');
Ja_inv(isnan(Ja_inv)) = 0;

% Matrices
S = get_CoriolisMatrix(q,q_dot);
tau_fric = get_FrictionTorque(q_dot);
G = get_GravityVector(q);
I = eye(6);

% Impedance controller (De Luca)
%{
Bx = (Ja_inv')* B * Ja_inv;
tau = B*Ja_inv*(ddzdes - Ja_dot*q_dot + ...
    inv(Bm)*(Dm*(dzdes - dz) + Km*(zdes- z))) + S*q_dot + tau_fric + G + ...
    (Ja')*(Bx*inv(Bm) - I)*F_ext;
%}
% Impedance controller (Albu Shaffer)
B_inv = inv(B)
L = inv(Ja * B_inv * Ja');
L(isnan(L)) = 0;
e_pos = (z - zdes);
e_pos_dot = (dz - dzdes);
e_or = zeros(3,1);
%e_or = (or - or_des);
e_or = wrapToPi(or-or_des);
e_or_dot = Ja(4:6,1:7)*q_dot;
e = [e_pos; e_or];
e_dot = [e_pos_dot; e_or_dot];                                                                   
a_des = [ddzdes; zeros(3,1)];
F_tau = L*a_des - L*inv(Bm)*(Dm*e_dot + Km*e) + (L*inv(Bm) - I)*F_ext - L*Ja_dot*q_dot;
tau = (Ja')*F_tau + S*q_dot + tau_fric + G;

end

== matlab function tests_control_franka/FRANKA_Model_Joint_Space2/CORIOLIS ==
  data: q input; Fc output double; q_dot input
function Fc = fcn(q,q_dot)
coder.extrinsic('get_CoriolisMatrix');
C = zeros(7,7);
C = get_CoriolisMatrix(q,q_dot);

Fc = C*q_dot;

end

== matlab function tests_control_franka/FRANKA_Model_Joint_Space2/GRAVITY ==
  data: q input; G output double
function G = fcn(q)
coder.extrinsic('get_GravityVector');
G = zeros(7,1);
G = get_GravityVector(q);

end

== matlab function tests_control_franka/FRANKA_Model_Joint_Space2/Joint Friction ==
  data: q_dot input; tau_f output
function tau_f = fcn(q_dot)
coder.extrinsic('get_FrictionTorque');
tau_f = zeros(7,1);
tau_f = get_FrictionTorque(q_dot);

end

== matlab function tests_control_franka/FRANKA_Model_Joint_Space2/Joint Friction1 ==
  data: q_dot input; tau_f output
function tau_f = fcn(q_dot)
D=eye(7)*1;
tau_f = -D*q_dot;

end

== matlab function tests_control_franka/FRANKA_Model_Joint_Space2/MASS^-1 ==
  data: q input; ddq output; F_tot input double
function ddq = fcn(q,F_tot)
coder.extrinsic('get_MassMatrix');
B = zeros(7,7);
B = get_MassMatrix(q);
B(isnan(B)) = 0;
cond_B = cond(B)

ddq = B\F_tot;                      % Ftot*M^-1

end

== matlab function tests_control_franka/FRANKA_Model_Joint_Space2/MATLAB Function ==
  data: F input; F_ext output double; q input
function F_ext = fcn(F,q)
coder.extrinsic('get_Ja');
Ja = zeros(6,7);
Ja = get_Ja(q);

F_ext = zeros(7,1);
F_ext = (Ja')*F;

end

== matlab function tests_control_franka/PLANNER2/KY_GENERATOR ==
  settings: updateMethod=DISCRETE  sampleTime=Ts
  data: k output; F_ext input; z input; z_des input; dz_des input; int input; comp input; e_max parameter; F_max parameter; F_int_max parameter
function k = fcn(F_ext, z, z_des, dz_des, int, comp, e_max, F_max, F_int_max)
%% Description
% Set the K coefficient for a variable impedance controller based on a
% desired trajectory

%% Outputs
% k             stiffness

%% Inputs
% F_ext         measured external force
% z_des         desired trajectory
% z             current position
% int, comp     booleans for the interaction and compensation phase

%% Parameters
% F_int_max     desired interaction force
% F_max         nominal disturbance forces
% e_max         maximum steady-state error

%% persistent initialization
persistent ki kc F_comp int_prec comp_prec z_int z_int_dir set_F_comp
if isempty(ki)
   ki = F_max/e_max;        % k obtained from interaction
end
if isempty(F_comp)
   F_comp = 0;              % weight to compensate
end
if isempty(kc)
      kc = F_max/e_max;     % k obtained from compensation
end
if isempty(z_int) 
    z_int = 1000;       % obstacle(or interaction) position
end
if isempty(z_int_dir) 
    z_int_dir = 0;          % prohibited direction due to the obstacle
end
if isempty(int_prec)
    int_prec = 0;           % previous values of int
end
if isempty(comp_prec)
    comp_prec = 0;          % previous values od comp
end
if isempty(set_F_comp)
    set_F_comp = 1;
end
%% INTERACTION
% set ki in order to match a desired interaction force with the
% envirorment, and store interaction's position when detected
% X axes
if int == 1
    % detection of an interaction 
    if abs(F_ext-F_comp) > F_max
        if z_int == 1000                     % z_int has not been set yet
            z_int = z;
            z_int_dir = -sign(F_ext-F_comp);
            set_F_comp = 0; 
        end
    end
    % setting of ki
    if abs(F_ext-F_comp) > F_int_max 
        % if interaction force is higher than threshold
        if ki*abs(z-z_des) > F_int_max
            ktemp_x = F_int_max/abs(z-z_des);
            if ktemp_x < ki                % ki needs to be only decreased
                ki = ktemp_x;
            end
        end
    end
end

%% COMPENSATION
% set kc in order to compensate the effect of the weight of the object,
% and store it
% X axes
if comp == 1
    % compensation detection
    if z_int == 1000                     % z_int not set before
        if abs(F_ext)/kc > e_max         
            kc = abs(F_ext)/e_max;
            if set_F_comp > 0.1
                F_comp = F_ext;
            end
        end
    else 
        if z_int_dir == 1                % obstacle in above
            if z < z_int
                if abs(F_ext)/kc > e_max 
                    kc = abs(F_ext)/e_max;
                    if set_F_comp > 0.1
                        F_comp = F_ext;
                    end
                end
            end
        else                                % obstacle is below
            if z > z_int
                if abs(F_ext)/kc > e_max
                    kc = abs(F_ext)/e_max;
                    if set_F_comp > 0.1
                        F_comp = F_ext;
                    end
                end
            end
        end 
   end
end

%% reset to default values when comp or int shifts to zero
if comp==0 && comp_prec==1
    kc = F_max/e_max;
    F_comp = 0;
    set_F_comp = 0;
end
if int==0 && int_prec==1
    ki = F_max/e_max;
end

%% from int to comp and vice versa
if int==1 && int_prec==0
    if comp_prec == 1
        ki = kc;
    end
    z_int=1000;
    z_int_dir=0;
end
if comp == 1 && comp_prec==0
    if int_prec == 1
        kc = ki;
    end
    set_F_comp = 1;
end

% update to last booleans
int_prec = int;
comp_prec = comp;


%% Selection of Final Values of D-K
% default values
k = abs(F_max)/e_max;

% compensation
if comp == 1
    k = kc;
end

% both compensation and interaction are activated
% if "away" from obstacle set k = kc else ki
if int == 1
    k = ki;
    if comp == 1
        if z_int == 1000
            k = kc;                       % obstacle not reached
        else
            if z_int_dir == 1
                if z_des < z_int
                    if sign(dz_des*z_int_dir) < 0
                        k = kc;               % obstacle reached but "going away"
                    end
                end
            else
                if z_des > z_int
                    if sign(dz_des*z_int_dir) < 0
                        k = kc;               % obstacle reached but "going away"
                    end
                end
            end
        end
    else
        if z_int == 1000
            k = F_max/e_max;            % restore to default
        else
            if z_int_dir == 1
                if z_des < z_int
                    k = F_max/e_max;    % restore because "going away"
                end
            else
                if z_des > z_int
                    k = F_max/e_max;    % restore because "going away"
                end
            end
        end
    end
end

end

== matlab function tests_control_franka/TRAJECTORY1/GENERATOR ==
  data: time input; z_des output; dz_des output; ddz_des output; or_des output; int output; comp output
function  [z_des, dz_des, ddz_des, or_des, int, comp] = fcn(time)
coder.extrinsic('wrapToPi')
t= time;
int = [0; 0; 0];
comp = [0; 0; 0];
q = [0; pi/4; 0; -pi/2; 0; 0; 0];
or_init = zeros(3,1);
or_init = wrapToPi([-3.14;0.78+pi/4;0]);
pos_init = [0.35; 0; 0.3];
or_des = or_init;
or_des = wrapToPi(or_des);

z_des = pos_init + [0; cos(2*t)/8; sin(2*t)/8];
dz_des = [0; -sin(2*t)/4; cos(2*t)/4];
ddz_des = [0; -cos(2*t)/2; -sin(2*t)/2];

end

== matlab function tests_control_franka/PLANNER2/KD_INTERPOLATOR  ==
  settings: updateMethod=DISCRETE  sampleTime=Ts
  data: time input; K output; kx_f input; ky_f input; kz_f input; D output; e_max parameter; F_max parameter; M parameter; berta parameter; a0 parameter; mass parameter; csi parameter; Kvis output; Dvis output
function [K,D,Kvis, Dvis] = fcn(time, kx_f, ky_f, kz_f, e_max, F_max, M, berta, a0, mass, csi)
%% Description
% Interpolate K in order to guarantee stability

%% Outputs
% K             Stiffness matrix
% D             Damping matrix

%% Inputs
% kx_f, ky, f   desired values of K

%% Parameters
% F_max         nominal disturbance forces
% e_max         maximum steady-state error
% M             virtual mass
% berta, a0     parameters for the computation of stability conditions
% mass          virtual mass

%% persistent initialization
persistent kx ky kz time_prec
if isempty(time_prec)
    time_prec = 0;              % previous simulation time
end
if isempty(kx)
   kx = F_max/e_max;         % last value of k
end
if isempty(ky)
   ky = F_max/e_max;
end
if isempty(kz)
   kz = F_max/e_max;
end

% set k from desired one 
if kx_f <= kx       
    kx = kx_f;
else 
    % increese k in accordance with the stability conditions
    kx_i = kx;
    k_dotx = berta*(4*a0*sqrt(kx_i/mass)*(kx_i)^(3/2))/(sqrt(kx_i) + 2*a0*csi*sqrt(kx_i));
    k_tempx = kx_i + k_dotx*(time -time_prec);
    if k_tempx > kx_f
        kx = kx_f;
    else
        kx = k_tempx;
    end
end

% Y axes, same as X axes
if ky_f <= ky
    ky = ky_f;
else 
    ky_i = ky;
    k_doty = berta*(4*a0*sqrt(ky_i/mass)*(ky_i)^(3/2))/(sqrt(ky_i) + 2*a0*csi*sqrt(ky_i));
    k_tempy = ky_i + k_doty*(time -time_prec);
    if k_tempy > ky_f
        ky = ky_f;
    else
        ky = k_tempy;
    end
end

% Z axes, same as other axes
if kz_f <= kz
    kz = kz_f;
else 
    kz_i = kz;
    k_dotz = berta*(4*a0*sqrt(kz_i/mass)*(kz_i)^(3/2))/(sqrt(kz_i) + 2*a0*csi*sqrt(kz_i));
    k_tempz = kz_i + k_dotz*(time -time_prec);
    if k_tempz > kz_f
        kz = kz_f;
    else
        kz = k_tempz;
    end
end

time_prec = time;

% damping computation, critically damped condition
dx = sqrt(4*kx*M);
dy = sqrt(4*ky*M);
dz = sqrt(4*kz*M);

%% Final impedance matrices
D = zeros(6,6);
K = zeros(6,6);
D(1:3,1:3) = diag([dx, dy, dz]);
D(4:6,4:6) = diag([2*sqrt(300) 2*sqrt(300) 2*sqrt(300)]); %rot damping
K(1:3,1:3) = diag([kx, ky, kz]);
K(4:6,4:6) = diag ([300 300 300]); %rot stiffness
Kvis = [kx; ky; kz];
Dvis = [dx; dy; dz];
end
